simulink model "sdbe_8_11"  (R2012b)
settings: Solver=VariableStepDiscrete  SolverMode=SingleTasking  StartTime=0.0  StopTime=10000  RelTol=1e-3
PreLoadFcn:
  | counter_vals
undefined symbols (not defined in the file or in its folder): sfp
libraries: xbsIndex_r4 x6687, casper_library_misc x35, casper_library_delays x27, dspsigops x16, xps_library x10, r2dbe_vdif_lib x4, r2dbe_adc_lib x3, simulink x1
(part 1 of 58)
settings Model: Creator=lvertats  LastModifiedBy=lvertats
settings OptimizationCC: InlineParams=on

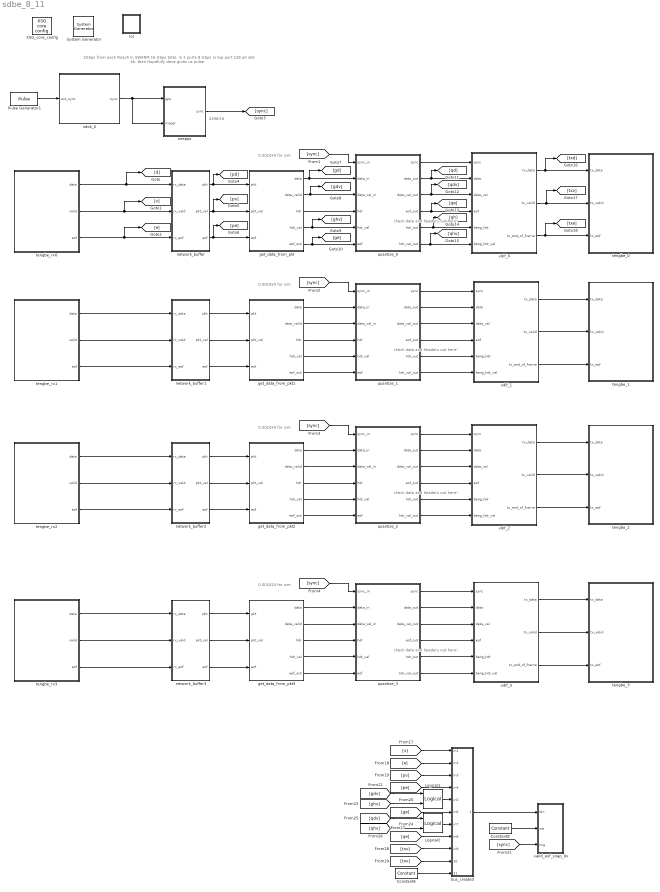
== system sdbe_8_11 ==
  note: 0.001024 for sim
  note: 2496/16
  note: check data and headers out here!
  note: 2Gbps from each Roach in SWARM
      | 16 Gbps total, in 2 ports
      | 8 Gbps in top port
      | 128 p0 sb0 4b, then
      |
      | Hopefully dave gives us pulse
  note: 0.001024 for sim
  note: check data and headers out here!
  note: 0.001024 for sim
  note: check data and headers out here!
  note: 0.001024 for sim
  note: check data and headers out here!
  " System Generator" : xbsIndex_r4/ System Generator  Tag=genX  xilinxfamily=virtex6  part=xc6vsx475t  speed=-1  package=ff1759  synthesis_tool=XST  clock_wrapper=Clock Enables  directory=./sdbe_8_11/sysgen  proj_type=Project Navigator  Synth_file=XST Defaults  Impl_file=ISE Defaults  testbench=off  simulink_period=1  sysclk_period=4.8077  dcm_input_clock_period=100  incr_netlist=off  trim_vbits=Everywhere in SubSystem  dbl_ovrd=According to Block Masks  core_generation=According to Block Masks  run_coregen=off  deprecated_control=off  eval_field=0  block_type=sysgen
  Constant6 : xbsIndex_r4/Constant  const=0  gui_display_data_type=Fixed-point  arith_type=Unsigned  n_bits=6  bin_pt=0  preci_type=Single  exp_width=8  frac_width=24  explicit_period=on  period=1  equ=P=C  opselect=C  inp2=PCIN>>17  opr=+  inp1=P  carry=CIN  dbl_ovrd=off  block_type=constant
  Constant8 : xbsIndex_r4/Constant  const=1  gui_display_data_type=Boolean  arith_type=Boolean  n_bits=31  bin_pt=0  preci_type=Single  exp_width=8  frac_width=24  explicit_period=on  period=1  equ=P=C  opselect=C  inp2=PCIN>>17  opr=+  inp1=P  carry=CIN  dbl_ovrd=off  block_type=constant
  Logical1 : xbsIndex_r4/Logical  logical_function=OR  inputs=2  en=off  latency=0  precision=Full  arith_type=Unsigned  n_bits=16  bin_pt=0  align_bp=on  dbl_ovrd=off  block_type=logical
  Logical2 : xbsIndex_r4/Logical  logical_function=OR  inputs=2  en=off  latency=0  precision=Full  arith_type=Unsigned  n_bits=16  bin_pt=0  align_bp=on  dbl_ovrd=off  block_type=logical
  Pulse Generator1 : DiscretePulseGenerator  Period=1024  PhaseDelay=57
  XSG_core_config : xps_library/XSG core config  Tag=xps:xsg  hw_sys=ROACH2:sx475t  clk_src=adc0_clk  ROACH_clk_src=sys_clk  ROACH2_clk_src=adc0_clk  MKDIG_clk_src=sys_clk  clk_rate=3328/16  sample_period=1  synthesis_tool=XST
  bus_create3 : Subsystem  AncestorBlock=casper_library_flow_control/bus_create  mask(bus_create){inputNum=11}
      mask prompts: inputNum "Number of inputs:"
      mask init:
      | bus_create_init(gcb,...
      |     'inputNum', inputNum);
  get_data_from_pkt : Subsystem
  get_data_from_pkt1 : Subsystem
  get_data_from_pkt2 : Subsystem
  get_data_from_pkt3 : Subsystem
  network_buffer : Subsystem
  network_buffer1 : Subsystem
  network_buffer2 : Subsystem
  network_buffer3 : Subsystem
  onepps : Subsystem  AncestorBlock=r2dbe_adc_lib/onepps  mask(r2dbe_onepps){clk_rate=3328/16}
      mask prompts: clk_rate "FPGA clock rate (MHz):"
      mask help: Sub-system for 1pps parameters of the R2DBE.
  quantize_0 : Subsystem  mask(r2dbe_quantize){mult_delay=3, add_delay=2, convert_delay=1, pipeline_delay=1, io_delay=3}
      mask prompts: mult_delay "Multiplier latency:"; add_delay "Adder latency:"; convert_delay "Convert latency:"; pipeline_delay "Output pipeline delay:"; io_delay "I/O delay:"
      mask help: Sub-system for quantization parameters of the R2DBE.
  quantize_1 : Subsystem  mask(r2dbe_quantize){mult_delay=3, add_delay=2, convert_delay=1, pipeline_delay=1, io_delay=3}
      mask prompts: mult_delay "Multiplier latency:"; add_delay "Adder latency:"; convert_delay "Convert latency:"; pipeline_delay "Output pipeline delay:"; io_delay "I/O delay:"
      mask help: Sub-system for quantization parameters of the R2DBE.
  quantize_2 : Subsystem  mask(r2dbe_quantize){mult_delay=3, add_delay=2, convert_delay=1, pipeline_delay=1, io_delay=3}
      mask prompts: mult_delay "Multiplier latency:"; add_delay "Adder latency:"; convert_delay "Convert latency:"; pipeline_delay "Output pipeline delay:"; io_delay "I/O delay:"
      mask help: Sub-system for quantization parameters of the R2DBE.
  quantize_3 : Subsystem  mask(r2dbe_quantize){mult_delay=3, add_delay=2, convert_delay=1, pipeline_delay=1, io_delay=3}
      mask prompts: mult_delay "Multiplier latency:"; add_delay "Adder latency:"; convert_delay "Convert latency:"; pipeline_delay "Output pipeline delay:"; io_delay "I/O delay:"
      mask help: Sub-system for quantization parameters of the R2DBE.
  rcs : Subsystem  AncestorBlock=casper_library_misc/rcs  mask(rcs){app_src=timestamp, lib_src=timestamp, user_val=0}
      mask prompts: app_src "Application revision info to capture"; lib_src "CASPER libraries revision info to capture"; user_val "User specified value"
      mask help:
      | Embeds revision control information for the user design and libraries.
      | On failure to locate specified revision information, falls back to
      | timestamps (current time for libraries).
      | A user specified value is also stored.
      mask init:
      | rcs_init(gcb, ...
      |     'app_src', app_src, ...
      |     'lib_src', lib_src);
      mask TypeOptions app_src: timestamp | git | svn
      mask TypeOptions lib_src: timestamp | git | svn
  tengbe_0 : Subsystem  mask(r2dbe_tengbe){slot=0, port=0}
      mask prompts: slot "Card slot:"
      mask help: Sub-system for 10 GbE parameters of the R2DBE.
      mask init:
      | set_param([gcb, '/core'], 'slot', slot);
      | set_param([gcb, '/core'], 'port_r2_sfpp', port);
      mask TypeOptions slot: 0 | 1
      mask TypeOptions port: 0 | 1 | 2 | 3
  tengbe_1 : Subsystem  mask(r2dbe_tengbe){slot=0, port=1}
      mask prompts: slot "Card slot:"
      mask help: Sub-system for 10 GbE parameters of the R2DBE.
      mask init:
      | set_param([gcb, '/core'], 'slot', slot);
      | set_param([gcb, '/core'], 'port_r2_sfpp', port);
      mask TypeOptions slot: 0 | 1
      mask TypeOptions port: 0 | 1 | 2 | 3
  tengbe_2 : Subsystem  mask(r2dbe_tengbe){slot=0, port=2}
      mask prompts: slot "Card slot:"
      mask help: Sub-system for 10 GbE parameters of the R2DBE.
      mask init:
      | set_param([gcb, '/core'], 'slot', slot);
      | set_param([gcb, '/core'], 'port_r2_sfpp', port);
      mask TypeOptions slot: 0 | 1
      mask TypeOptions port: 0 | 1 | 2 | 3
  tengbe_3 : Subsystem  mask(r2dbe_tengbe){slot=0, port=3}
      mask prompts: slot "Card slot:"
      mask help: Sub-system for 10 GbE parameters of the R2DBE.
      mask init:
      | set_param([gcb, '/core'], 'slot', slot);
      | set_param([gcb, '/core'], 'port_r2_sfpp', port);
      mask TypeOptions slot: 0 | 1
      mask TypeOptions port: 0 | 1 | 2 | 3
  tengbe_rx0 : Subsystem  mask(r2dbe_tengbe){slot=1, port=0}
      mask prompts: slot "Card slot:"
      mask help: Sub-system for 10 GbE parameters of the R2DBE.
      mask init:
      | set_param([gcb, '/core'], 'slot', slot);
      | set_param([gcb, '/core'], 'port_r2_sfpp', port);
      mask TypeOptions slot: 0 | 1
      mask TypeOptions port: 0 | 1 | 2 | 3
  tengbe_rx1 : Subsystem  mask(r2dbe_tengbe){slot=1, port=1}
      mask prompts: slot "Card slot:"
      mask help: Sub-system for 10 GbE parameters of the R2DBE.
      mask init:
      | set_param([gcb, '/core'], 'slot', slot);
      | set_param([gcb, '/core'], 'port_r2_sfpp', port);
      mask TypeOptions slot: 0 | 1
      mask TypeOptions port: 0 | 1 | 2 | 3
  tengbe_rx2 : Subsystem  mask(r2dbe_tengbe){slot=1, port=2}
      mask prompts: slot "Card slot:"
      mask help: Sub-system for 10 GbE parameters of the R2DBE.
      mask init:
      | set_param([gcb, '/core'], 'slot', slot);
      | set_param([gcb, '/core'], 'port_r2_sfpp', port);
      mask TypeOptions slot: 0 | 1
      mask TypeOptions port: 0 | 1 | 2 | 3
  tengbe_rx3 : Subsystem  mask(r2dbe_tengbe){slot=1, port=3}
      mask prompts: slot "Card slot:"
      mask help: Sub-system for 10 GbE parameters of the R2DBE.
      mask init:
      | set_param([gcb, '/core'], 'slot', slot);
      | set_param([gcb, '/core'], 'port_r2_sfpp', port);
      mask TypeOptions slot: 0 | 1
      mask TypeOptions port: 0 | 1 | 2 | 3
  valid_eof_snap_0x : Subsystem  Tag=casper:snapshot  AncestorBlock=casper_library_scopes/snapshot  mask(snapshot){storage=bram, dram_dimm=1, dram_clock=200, nsamples=14, data_width=16, offset=off, circap=off, value=off, use_dsp48=on}
      mask prompts: storage "Storage medium"; dram_dimm "DRAM dimm"; dram_clock "DRAM clock rate"; nsamples "Number of Samples (2^?)"; data_width "Data width"; offset "Start delay support"; circap "Circular capture support"; value "Extra value capture support"; use_dsp48 "Use DSP48s to implement counters"
      mask help:
      | Standard snap block, but with the following optional extras;
      |  1) Optionally delay the fabric trigger by a user-specified number of valids.
      |  2) Capture continuously after a trigger until a stop pulse is received. Data is captured into BRAM continuously, with old data being overwritten until a stop command is received. Then stop capturing when memory is filled. This enables you to get some data before and some data after the stop pulse. Use the 'tr_en_cnt' register to determine where you are in your vector. 'Addr' register's MSb now indicates 'busy capturing'.
      |  3) Optionally capture a value on an input port to a register at the same time as the first data sample.
      |  4) Implement counters using DSP48Es to save resources.
      mask init:
      | snapshot_init(gcb, ...
      |     'storage', storage, ...
      |     'dram_dimm', dram_dimm, ...
      |     'dram_clock', dram_clock, ...
      |     'nsamples', nsamples, ...
      |     'data_width', data_width, ...
      |     'offset', offset, ...
      |     'circap', circap, ...
      |     'value', value, ...
      |     'use_dsp48', use_dsp48);
      mask TypeOptions storage: bram | dram
      mask Callback storage: snapshot_callback();
      mask TypeOptions dram_dimm: 1 | 2 | 3 | 4
      mask TypeOptions dram_clock: 200 | 250 | 266 | 300 | 333
      mask TypeOptions data_width: 8 | 16 | 32 | 64 | 128
  vdif_0 : Subsystem  mask(r2dbe_vdif){}
      mask help: Sub-system for VDIF parameters of the R2DBE.
  vdif_1 : Subsystem  mask(r2dbe_vdif){}
      mask help: Sub-system for VDIF parameters of the R2DBE.
  vdif_2 : Subsystem  mask(r2dbe_vdif){}
      mask help: Sub-system for VDIF parameters of the R2DBE.
  vdif_3 : Subsystem  mask(r2dbe_vdif){}
      mask help: Sub-system for VDIF parameters of the R2DBE.
  zdok_0 : Subsystem  mask(r2dbe_zdok){zdok=ZDOK 0, nyquist_bw=1248, pipeline_delay=1}
      mask prompts: zdok "ADC board"; nyquist_bw "Nyquist bandwidth (MHz):"; pipeline_delay "Output pipeline delay:"
      mask help: Sub-system for ADC5g parameters of the R2DBE.
      mask init:
      | set_param([gcb, '/adc'], 'adc_brd', zdok);
      mask TypeOptions zdok: ZDOK 0 | ZDOK 1
  wires:
  vdif_0/1(tx_data) -> tengbe_0/1(tx_data), [txd]
  vdif_0/2(tx_valid) -> tengbe_0/2(tx_valid), [txv]
  vdif_0/3(tx_end_of_frame) -> [txe], tengbe_0/3(tx_eof)
  quantize_0/1(sync) -> vdif_0/1(sync)
  quantize_0/2(data_out) -> vdif_0/2(data), [qd]
  Pulse Generator1/1 -> zdok_0/1(ext_sync)
  zdok_0/1(sync) -> onepps/2(maser), onepps/1(gps)
  onepps/1(sync) -> [sync]
  quantize_0/3(data_val_out) -> vdif_0/3(data_val), [qdv]
  quantize_0/4(eof_out) -> vdif_0/4(eof), [qe]
  quantize_0/5(hdr_out) -> vdif_0/5(beng_hdr), [qh]
  quantize_0/6(hdr_val_out) -> vdif_0/6(beng_hdr_val), [qhv]
  network_buffer/1(pkt) -> [pd], get_data_from_pkt/1(pkt)
  network_buffer/2(pkt_val) -> [pv], get_data_from_pkt/2(pkt_val)
  network_buffer/3(eof) -> [pe], get_data_from_pkt/3(eof)
  get_data_from_pkt/5(eof_out) -> [ge], quantize_0/6(eof)
  get_data_from_pkt/4(hdr_val) -> [ghv], quantize_0/5(hdr_val)
  get_data_from_pkt/3(hdr) -> quantize_0/4(hdr)
  get_data_from_pkt/2(data_valid) -> [gdv], quantize_0/3(data_val_in)
  get_data_from_pkt/1(data) -> [gd], quantize_0/2(data_in)
  bus_create3/1(bus_out) -> valid_eof_snap_0x/1(din)
  Constant8/1 -> valid_eof_snap_0x/2(we)
  [sync] -> valid_eof_snap_0x/3(trig)
  [e] -> bus_create3/2(in2)
  [v] -> bus_create3/1(in1)
  [pv] -> bus_create3/3(in3)
  [pe] -> bus_create3/4(in4)
  Logical1/1 -> bus_create3/5(in5)
  [gdv] -> Logical1/1
  [ghv] -> Logical1/2
  [ge] -> bus_create3/6(in6)
  [qdv] -> Logical2/1
  [qhv] -> Logical2/2
  [qe] -> bus_create3/8(in8)
  Logical2/1 -> bus_create3/7(in7)
  [txv] -> bus_create3/9(in9)
  [txv] -> bus_create3/10(in10)
  Constant6/1 -> bus_create3/11(in11)
  tengbe_rx0/1(data) -> [d], network_buffer/1(rx_data)
  tengbe_rx0/2(valid) -> [v], network_buffer/2(rx_vald)
  tengbe_rx0/3(eof) -> [e], network_buffer/3(rx_eof)
  [sync] -> quantize_0/1(sync_in)
  quantize_1/1(sync) -> vdif_1/1(sync)
  quantize_1/2(data_out) -> vdif_1/2(data)
  quantize_1/3(data_val_out) -> vdif_1/3(data_val)
  quantize_1/4(eof_out) -> vdif_1/4(eof)
  quantize_1/5(hdr_out) -> vdif_1/5(beng_hdr)
  quantize_1/6(hdr_val_out) -> vdif_1/6(beng_hdr_val)
  network_buffer1/1(pkt) -> get_data_from_pkt1/1(pkt)
  network_buffer1/2(pkt_val) -> get_data_from_pkt1/2(pkt_val)
  network_buffer1/3(eof) -> get_data_from_pkt1/3(eof)
  get_data_from_pkt1/5(eof_out) -> quantize_1/6(eof)
  get_data_from_pkt1/4(hdr_val) -> quantize_1/5(hdr_val)
  get_data_from_pkt1/3(hdr) -> quantize_1/4(hdr)
  get_data_from_pkt1/2(data_valid) -> quantize_1/3(data_val_in)
  get_data_from_pkt1/1(data) -> quantize_1/2(data_in)
  tengbe_rx1/1(data) -> network_buffer1/1(rx_data)
  tengbe_rx1/2(valid) -> network_buffer1/2(rx_vald)
  tengbe_rx1/3(eof) -> network_buffer1/3(rx_eof)
  [sync] -> quantize_1/1(sync_in)
  quantize_2/1(sync) -> vdif_2/1(sync)
  quantize_2/2(data_out) -> vdif_2/2(data)
  quantize_2/3(data_val_out) -> vdif_2/3(data_val)
  quantize_2/4(eof_out) -> vdif_2/4(eof)
  quantize_2/5(hdr_out) -> vdif_2/5(beng_hdr)
  quantize_2/6(hdr_val_out) -> vdif_2/6(beng_hdr_val)
  network_buffer2/1(pkt) -> get_data_from_pkt2/1(pkt)
  network_buffer2/2(pkt_val) -> get_data_from_pkt2/2(pkt_val)
  network_buffer2/3(eof) -> get_data_from_pkt2/3(eof)
  get_data_from_pkt2/5(eof_out) -> quantize_2/6(eof)
  get_data_from_pkt2/4(hdr_val) -> quantize_2/5(hdr_val)
  get_data_from_pkt2/3(hdr) -> quantize_2/4(hdr)
  get_data_from_pkt2/2(data_valid) -> quantize_2/3(data_val_in)
  get_data_from_pkt2/1(data) -> quantize_2/2(data_in)
  tengbe_rx2/1(data) -> network_buffer2/1(rx_data)
  tengbe_rx2/2(valid) -> network_buffer2/2(rx_vald)
  tengbe_rx2/3(eof) -> network_buffer2/3(rx_eof)
  [sync] -> quantize_2/1(sync_in)
  quantize_3/1(sync) -> vdif_3/1(sync)
  quantize_3/2(data_out) -> vdif_3/2(data)
  quantize_3/3(data_val_out) -> vdif_3/3(data_val)
  quantize_3/4(eof_out) -> vdif_3/4(eof)
  quantize_3/5(hdr_out) -> vdif_3/5(beng_hdr)
  quantize_3/6(hdr_val_out) -> vdif_3/6(beng_hdr_val)
  network_buffer3/1(pkt) -> get_data_from_pkt3/1(pkt)
  network_buffer3/2(pkt_val) -> get_data_from_pkt3/2(pkt_val)
  network_buffer3/3(eof) -> get_data_from_pkt3/3(eof)
  get_data_from_pkt3/5(eof_out) -> quantize_3/6(eof)
  get_data_from_pkt3/4(hdr_val) -> quantize_3/5(hdr_val)
  get_data_from_pkt3/3(hdr) -> quantize_3/4(hdr)
  get_data_from_pkt3/2(data_valid) -> quantize_3/3(data_val_in)
  get_data_from_pkt3/1(data) -> quantize_3/2(data_in)
  tengbe_rx3/1(data) -> network_buffer3/1(rx_data)
  tengbe_rx3/2(valid) -> network_buffer3/2(rx_vald)
  tengbe_rx3/3(eof) -> network_buffer3/3(rx_eof)
  [sync] -> quantize_3/1(sync_in)
  vdif_1/3(tx_end_of_frame) -> tengbe_1/3(tx_eof)
  vdif_1/1(tx_data) -> tengbe_1/1(tx_data)
  vdif_1/2(tx_valid) -> tengbe_1/2(tx_valid)
  vdif_2/2(tx_valid) -> tengbe_2/2(tx_valid)
  vdif_2/3(tx_end_of_frame) -> tengbe_2/3(tx_eof)
  vdif_2/1(tx_data) -> tengbe_2/1(tx_data)
  vdif_3/2(tx_valid) -> tengbe_3/2(tx_valid)
  vdif_3/3(tx_end_of_frame) -> tengbe_3/3(tx_eof)
  vdif_3/1(tx_data) -> tengbe_3/1(tx_data)

== system sdbe_8_11/bus_create3 ==
  in1 : Inport
  in2 : Inport  Port=2
  in3 : Inport  Port=3
  in4 : Inport  Port=4
  in5 : Inport  Port=5
  in6 : Inport  Port=6
  in7 : Inport  Port=7
  in8 : Inport  Port=8
  in9 : Inport  Port=9
  in10 : Inport  Port=10
  in11 : Inport  Port=11
  concatenate : xbsIndex_r4/Concat  num_inputs=11  dbl_ovrd=off  block_type=concat
  reinterpret{1..11} (11 alike) : xbsIndex_r4/Reinterpret  force_arith_type=on  arith_type=Unsigned  force_bin_pt=on  bin_pt=0  block_type=reinterpret
      reinterpret1 settings: infoedit="Changes signal type without altering the binary representation.   You can changed the signal between signed and unsigned, and relocate the binary point.<br><br>Hardware notes: In hardware this block costs nothing.<br><br>Example:  Suppose the input is 6 bits wide, signed, with 2 fractional bits, and the output is forced to unsigned with 0 fractional bits.  Then an input of -2.0 (1110.00 in binary 2's complement) becomes an output of 56 (111000 in binary)."
      reinterpret2 settings: infoedit="Changes signal type without altering the binary representation.   You can changed the signal between signed and unsigned, and relocate the binary point.<br><br>Hardware notes: In hardware this block costs nothing.<br><br>Example:  Suppose the input is 6 bits wide, signed, with 2 fractional bits, and the output is forced to unsigned with 0 fractional bits.  Then an input of -2.0 (1110.00 in binary 2's complement) becomes an output of 56 (111000 in binary)."
  bus_out : Outport
  wires:
  concatenate/1 -> bus_out/1
  in1/1 -> reinterpret1/1
  reinterpret1/1 -> concatenate/1
  in2/1 -> reinterpret2/1
  reinterpret2/1 -> concatenate/2
  in3/1 -> reinterpret3/1
  reinterpret3/1 -> concatenate/3
  in4/1 -> reinterpret4/1
  reinterpret4/1 -> concatenate/4
  in5/1 -> reinterpret5/1
  reinterpret5/1 -> concatenate/5
  in6/1 -> reinterpret6/1
  reinterpret6/1 -> concatenate/6
  in7/1 -> reinterpret7/1
  reinterpret7/1 -> concatenate/7
  in8/1 -> reinterpret8/1
  reinterpret8/1 -> concatenate/8
  in9/1 -> reinterpret9/1
  reinterpret9/1 -> concatenate/9
  in10/1 -> reinterpret10/1
  reinterpret10/1 -> concatenate/10
  in11/1 -> reinterpret11/1
  reinterpret11/1 -> concatenate/11

== system sdbe_8_11/get_data_from_pkt ==
  note: can pass all through, but turn valid off for first
  pkt : Inport
  pkt_val : Inport  Port=2
  eof : Inport  Port=3
  Constant : Constant  Value=0
  Counter : xbsIndex_r4/Counter  cnt_type=Free Running  cnt_to=Inf  operation=Up  start_count=0  cnt_by_val=1  arith_type=Unsigned  n_bits=32  bin_pt=0  load_pin=off  rst=on  en=on  explicit_period=on  period=1  dbl_ovrd=off  use_behavioral_HDL=off  implementation=Fabric  block_type=counter
  Delay2 : xbsIndex_r4/Delay  rst=off  infoeditControl=Selection of Reset will increase slice count due to use of real FFs and instead of SRLs  en=off  latency=1  dbl_ovrd=off  reg_retiming=off  block_type=delay
  Delay3 : xbsIndex_r4/Delay  rst=off  infoeditControl=Selection of Reset will increase slice count due to use of real FFs and instead of SRLs  en=off  latency=1  dbl_ovrd=off  reg_retiming=off  block_type=delay
  Slice : xbsIndex_r4/Slice  nbits=1  boolean_output=on  mode=Upper Bit Location + Width  bit1=0  base1=MSB of Input  bit0=0  base0=LSB of Input  dbl_ovrd=off  block_type=slice
  Terminator : Terminator
  gen_valids1 : Subsystem
      mask help: latency 1
  npkts : Subsystem  Tag=xps:sw_reg  AncestorBlock=xps_library/software register  mask(swreg){mode=one value, io_dir=To Processor, io_delay=0, sample_period=1, names=reg, bitwidths=32, arith_types=0, bin_pts=0, sim_port=on, show_format=off}
      mask prompts: io_dir "I/O direction"; io_delay "I/O delay"; sample_period "Sample period"; names "Name:"; bitwidths "Bitwidth:"; arith_types "Type (ufix=0, fix=1, bool=2):"; bin_pts "Binary pt:"; sim_port "Provide sim input/output?"; show_format "Print format string?"
      mask init:
      | swreg_init(gcb)
      settings: AttributesFormatString=1output
      mask TypeOptions mode: one value | fields of equal size | fields of arbitrary size
      mask Callback mode: swreg_cb(gcb);
      mask TypeOptions io_dir: To Processor | From Processor
      mask Callback io_dir:
      | mask_enables = get_param(gcb, 'MaskEnables');
      | mask_names = get_param(gcb, 'MaskNames');
      | if strcmp(get_param(gcb, 'io_dir'), 'To Processor'),
      |     mask_enables{ismember(mask_names, 'sample_period')} = 'off';
      | else
      |     mask_enables{ismember(mask_names, 'sample_period')} = 'on';
      | end
      | set_param(gcb, 'MaskEnables', mask_enables);
      mask Callback bitwidths:
      | swreg_maskcheck(gcb);
      | % blk = gcb;
      | % mode = get_param(blk, 'mode');
      | % current_widths = eval(get_param(blk, 'bitwidths'));
      | % if (strcmp(mode, 'one value') || strcmp(mode, 'fields of equal size')) && (length(current_widths) > 1),
      | %     error('Only one width may be specified for this mode.');
      | % elseif strcmp(mode, 'fields of arbitrary size')
      | %     current_names = textscan(strtrim(strrep(strrep(get_param(blk, 'names'), ']', ''), '[', '')), '%s');
      | %     current_names = current_names{1};
      | %     numios = length(current_names);
      | %     if length(current_widths) ~= numios,
      | %         error('%d field names specified, but %d widths?', numios, length(current_widths));
      | %     end
      | % end
      | % total_width = 0;
      | % for ctr = 1 : length(current_widths),
      | %     total_width = total_width + current_widths(ctr);
      | % end
      | % if total_width > 32,
      | %     error('Total width must be 32 or less, set to %d.', total_width);
      | % end
      mask Callback arith_types:
      | [numios, ~, ~, ~, current_types] = swreg_maskcheck(gcb);
      | % blk = gcb;
      | % mode = get_param(blk, 'mode');
      | % current_types = eval(get_param(blk, 'arith_types'));
      | % numios = length(current_types);
      | % if (strcmp(mode, 'one value') || strcmp(mode, 'fields of equal size')) && (length(current_types) > 1),
      | %     error('Only one type may be specified for this mode.');
      | % elseif strcmp(mode, 'fields of arbitrary size')
      | %     current_names = textscan(strtrim(strrep(strrep(get_param(blk, 'names'), ']', ''), '[', '')), '%s');
      | %     current_names = current_names{1};
      | %     numios = length(current_names);
      | %     if length(current_types) ~= numios,
      | %         error('%d field names specified, but %d types?', numios, length(current_types));
      | %     end
      | % end
      | problem = 0;
      | for ctr = 1 : numios,
      |     t = current_types(ctr);
      |     if (t < 0) || (t > 2),
      |         problem = t;
      |         ctr = numios + 1;
      |     end
      | end
      | if problem ~= 0,
      |     error('Type cannot be %i, must be 0, 1 or 2.', problem);
      | end
      mask Callback bin_pts:
      | swreg_maskcheck(gcb);
      | % blk = gcb;
      | % mode = get_param(blk, 'mode');
      | % current_bins = eval(get_param(blk, 'bin_pts'));
      | % if (strcmp(mode, 'one value') || strcmp(mode, 'fields of equal size')) && (length(current_bins) > 1),
      | %     error('Only one binary pt may be specified for this mode.');
      | % elseif strcmp(mode, 'fields of arbitrary size')
      | %     current_names = textscan(strtrim(strrep(strrep(get_param(blk, 'names'), ']', ''), '[', '')), '%s');
      | %     current_names = current_names{1};
      | %     numios = length(current_names);
      | %     if length(current_bins) ~= numios,
      | %         error('%d field names specified, but %d binary pts?', numios, length(current_bins));
      | %     end
      | % end
  rst : Subsystem  Tag=xps:sw_reg  AncestorBlock=xps_library/software register  mask(swreg){mode=one value, io_dir=From Processor, io_delay=0, sample_period=1, names=reg, bitwidths=32, arith_types=0, bin_pts=0, sim_port=on, show_format=off}
      mask prompts: io_dir "I/O direction"; io_delay "I/O delay"; sample_period "Sample period"; names "Name:"; bitwidths "Bitwidth:"; arith_types "Type (ufix=0, fix=1, bool=2):"; bin_pts "Binary pt:"; sim_port "Provide sim input/output?"; show_format "Print format string?"
      mask init:
      | swreg_init(gcb)
      settings: AttributesFormatString=1input
      mask TypeOptions mode: one value | fields of equal size | fields of arbitrary size
      mask Callback mode: swreg_cb(gcb);
      mask TypeOptions io_dir: To Processor | From Processor
      mask Callback io_dir:
      | mask_enables = get_param(gcb, 'MaskEnables');
      | mask_names = get_param(gcb, 'MaskNames');
      | if strcmp(get_param(gcb, 'io_dir'), 'To Processor'),
      |     mask_enables{ismember(mask_names, 'sample_period')} = 'off';
      | else
      |     mask_enables{ismember(mask_names, 'sample_period')} = 'on';
      | end
      | set_param(gcb, 'MaskEnables', mask_enables);
      mask Callback bitwidths:
      | swreg_maskcheck(gcb);
      | % blk = gcb;
      | % mode = get_param(blk, 'mode');
      | % current_widths = eval(get_param(blk, 'bitwidths'));
      | % if (strcmp(mode, 'one value') || strcmp(mode, 'fields of equal size')) && (length(current_widths) > 1),
      | %     error('Only one width may be specified for this mode.');
      | % elseif strcmp(mode, 'fields of arbitrary size')
      | %     current_names = textscan(strtrim(strrep(strrep(get_param(blk, 'names'), ']', ''), '[', '')), '%s');
      | %     current_names = current_names{1};
      | %     numios = length(current_names);
      | %     if length(current_widths) ~= numios,
      | %         error('%d field names specified, but %d widths?', numios, length(current_widths));
      | %     end
      | % end
      | % total_width = 0;
      | % for ctr = 1 : length(current_widths),
      | %     total_width = total_width + current_widths(ctr);
      | % end
      | % if total_width > 32,
      | %     error('Total width must be 32 or less, set to %d.', total_width);
      | % end
      mask Callback arith_types:
      | [numios, ~, ~, ~, current_types] = swreg_maskcheck(gcb);
      | % blk = gcb;
      | % mode = get_param(blk, 'mode');
      | % current_types = eval(get_param(blk, 'arith_types'));
      | % numios = length(current_types);
      | % if (strcmp(mode, 'one value') || strcmp(mode, 'fields of equal size')) && (length(current_types) > 1),
      | %     error('Only one type may be specified for this mode.');
      | % elseif strcmp(mode, 'fields of arbitrary size')
      | %     current_names = textscan(strtrim(strrep(strrep(get_param(blk, 'names'), ']', ''), '[', '')), '%s');
      | %     current_names = current_names{1};
      | %     numios = length(current_names);
      | %     if length(current_types) ~= numios,
      | %         error('%d field names specified, but %d types?', numios, length(current_types));
      | %     end
      | % end
      | problem = 0;
      | for ctr = 1 : numios,
      |     t = current_types(ctr);
      |     if (t < 0) || (t > 2),
      |         problem = t;
      |         ctr = numios + 1;
      |     end
      | end
      | if problem ~= 0,
      |     error('Type cannot be %i, must be 0, 1 or 2.', problem);
      | end
      mask Callback bin_pts:
      | swreg_maskcheck(gcb);
      | % blk = gcb;
      | % mode = get_param(blk, 'mode');
      | % current_bins = eval(get_param(blk, 'bin_pts'));
      | % if (strcmp(mode, 'one value') || strcmp(mode, 'fields of equal size')) && (length(current_bins) > 1),
      | %     error('Only one binary pt may be specified for this mode.');
      | % elseif strcmp(mode, 'fields of arbitrary size')
      | %     current_names = textscan(strtrim(strrep(strrep(get_param(blk, 'names'), ']', ''), '[', '')), '%s');
      | %     current_names = current_names{1};
      | %     numios = length(current_names);
      | %     if length(current_bins) ~= numios,
      | %         error('%d field names specified, but %d binary pts?', numios, length(current_bins));
      | %     end
      | % end
  rx_output : Subsystem
  rx_output1 : Subsystem
  scope : Subsystem
  data : Outport
  data_valid : Outport  Port=2
  hdr : Outport  Port=3
  hdr_val : Outport  Port=4
  eof_out : Outport  Port=5
  wires:
  pkt/1 -> Delay2/1
  Delay2/1 -> [data], data/1, [hdr], hdr/1
  Delay3/1 -> [eof], eof_out/1
  eof/1 -> gen_valids1/2(eof), Delay3/1
  npkts/1(sim_out) -> Terminator/1
  Counter/1 -> npkts/1(out_reg)
  rst/1(in_reg) -> Slice/1
  Constant/1 -> rst/1(sim_1)
  Slice/1 -> Counter/1
  pkt_val/1 -> gen_valids1/1(pkt_val)
  gen_valids1/1(hdr_val) -> [hdr_val], hdr_val/1
  gen_valids1/2(data_val) -> [data_val], data_valid/1
  [eof] -> Counter/2
  [data_val] -> rx_output/2(val)
  [eof] -> rx_output/3(eof)
  [hdr_val] -> rx_output/1(sig)
  [data] -> rx_output1/3(data)
  [hdr] -> rx_output1/1(hdr)
  [hdr_val] -> rx_output1/2(hdr_val)
  [data_val] -> rx_output1/4(data_val)
  [data_val] -> scope/2(valid)
  [data] -> scope/1(data)

== system sdbe_8_11/get_data_from_pkt1 ==
  note: can pass all through, but turn valid off for first
  pkt : Inport
  pkt_val : Inport  Port=2
  eof : Inport  Port=3
  Constant : Constant  Value=0
  Counter : xbsIndex_r4/Counter  cnt_type=Free Running  cnt_to=Inf  operation=Up  start_count=0  cnt_by_val=1  arith_type=Unsigned  n_bits=32  bin_pt=0  load_pin=off  rst=on  en=on  explicit_period=on  period=1  dbl_ovrd=off  use_behavioral_HDL=off  implementation=Fabric  block_type=counter
  Delay2 : xbsIndex_r4/Delay  rst=off  infoeditControl=Selection of Reset will increase slice count due to use of real FFs and instead of SRLs  en=off  latency=1  dbl_ovrd=off  reg_retiming=off  block_type=delay
  Delay3 : xbsIndex_r4/Delay  rst=off  infoeditControl=Selection of Reset will increase slice count due to use of real FFs and instead of SRLs  en=off  latency=1  dbl_ovrd=off  reg_retiming=off  block_type=delay
  Slice : xbsIndex_r4/Slice  nbits=1  boolean_output=on  mode=Upper Bit Location + Width  bit1=0  base1=MSB of Input  bit0=0  base0=LSB of Input  dbl_ovrd=off  block_type=slice
  Terminator : Terminator
  gen_valids1 : Subsystem
      mask help: latency 1
  npkts : Subsystem  Tag=xps:sw_reg  AncestorBlock=xps_library/software register  mask(swreg){mode=one value, io_dir=To Processor, io_delay=0, sample_period=1, names=reg, bitwidths=32, arith_types=0, bin_pts=0, sim_port=on, show_format=off}
      mask prompts: io_dir "I/O direction"; io_delay "I/O delay"; sample_period "Sample period"; names "Name:"; bitwidths "Bitwidth:"; arith_types "Type (ufix=0, fix=1, bool=2):"; bin_pts "Binary pt:"; sim_port "Provide sim input/output?"; show_format "Print format string?"
      mask init:
      | swreg_init(gcb)
      settings: AttributesFormatString=1output
      mask TypeOptions mode: one value | fields of equal size | fields of arbitrary size
      mask Callback mode: swreg_cb(gcb);
      mask TypeOptions io_dir: To Processor | From Processor
      mask Callback io_dir:
      | mask_enables = get_param(gcb, 'MaskEnables');
      | mask_names = get_param(gcb, 'MaskNames');
      | if strcmp(get_param(gcb, 'io_dir'), 'To Processor'),
      |     mask_enables{ismember(mask_names, 'sample_period')} = 'off';
      | else
      |     mask_enables{ismember(mask_names, 'sample_period')} = 'on';
      | end
      | set_param(gcb, 'MaskEnables', mask_enables);
      mask Callback bitwidths:
      | swreg_maskcheck(gcb);
      | % blk = gcb;
      | % mode = get_param(blk, 'mode');
      | % current_widths = eval(get_param(blk, 'bitwidths'));
      | % if (strcmp(mode, 'one value') || strcmp(mode, 'fields of equal size')) && (length(current_widths) > 1),
      | %     error('Only one width may be specified for this mode.');
      | % elseif strcmp(mode, 'fields of arbitrary size')
      | %     current_names = textscan(strtrim(strrep(strrep(get_param(blk, 'names'), ']', ''), '[', '')), '%s');
      | %     current_names = current_names{1};
      | %     numios = length(current_names);
      | %     if length(current_widths) ~= numios,
      | %         error('%d field names specified, but %d widths?', numios, length(current_widths));
      | %     end
      | % end
      | % total_width = 0;
      | % for ctr = 1 : length(current_widths),
      | %     total_width = total_width + current_widths(ctr);
      | % end
      | % if total_width > 32,
      | %     error('Total width must be 32 or less, set to %d.', total_width);
      | % end
      mask Callback arith_types:
      | [numios, ~, ~, ~, current_types] = swreg_maskcheck(gcb);
      | % blk = gcb;
      | % mode = get_param(blk, 'mode');
      | % current_types = eval(get_param(blk, 'arith_types'));
      | % numios = length(current_types);
      | % if (strcmp(mode, 'one value') || strcmp(mode, 'fields of equal size')) && (length(current_types) > 1),
      | %     error('Only one type may be specified for this mode.');
      | % elseif strcmp(mode, 'fields of arbitrary size')
      | %     current_names = textscan(strtrim(strrep(strrep(get_param(blk, 'names'), ']', ''), '[', '')), '%s');
      | %     current_names = current_names{1};
      | %     numios = length(current_names);
      | %     if length(current_types) ~= numios,
      | %         error('%d field names specified, but %d types?', numios, length(current_types));
      | %     end
      | % end
      | problem = 0;
      | for ctr = 1 : numios,
      |     t = current_types(ctr);
      |     if (t < 0) || (t > 2),
      |         problem = t;
      |         ctr = numios + 1;
      |     end
      | end
      | if problem ~= 0,
      |     error('Type cannot be %i, must be 0, 1 or 2.', problem);
      | end
      mask Callback bin_pts:
      | swreg_maskcheck(gcb);
      | % blk = gcb;
      | % mode = get_param(blk, 'mode');
      | % current_bins = eval(get_param(blk, 'bin_pts'));
      | % if (strcmp(mode, 'one value') || strcmp(mode, 'fields of equal size')) && (length(current_bins) > 1),
      | %     error('Only one binary pt may be specified for this mode.');
      | % elseif strcmp(mode, 'fields of arbitrary size')
      | %     current_names = textscan(strtrim(strrep(strrep(get_param(blk, 'names'), ']', ''), '[', '')), '%s');
      | %     current_names = current_names{1};
      | %     numios = length(current_names);
      | %     if length(current_bins) ~= numios,
      | %         error('%d field names specified, but %d binary pts?', numios, length(current_bins));
      | %     end
      | % end
  rst : Subsystem  Tag=xps:sw_reg  AncestorBlock=xps_library/software register  mask(swreg){mode=one value, io_dir=From Processor, io_delay=0, sample_period=1, names=reg, bitwidths=32, arith_types=0, bin_pts=0, sim_port=on, show_format=off}
      mask prompts: io_dir "I/O direction"; io_delay "I/O delay"; sample_period "Sample period"; names "Name:"; bitwidths "Bitwidth:"; arith_types "Type (ufix=0, fix=1, bool=2):"; bin_pts "Binary pt:"; sim_port "Provide sim input/output?"; show_format "Print format string?"
      mask init:
      | swreg_init(gcb)
      settings: AttributesFormatString=1input
      mask TypeOptions mode: one value | fields of equal size | fields of arbitrary size
      mask Callback mode: swreg_cb(gcb);
      mask TypeOptions io_dir: To Processor | From Processor
      mask Callback io_dir:
      | mask_enables = get_param(gcb, 'MaskEnables');
      | mask_names = get_param(gcb, 'MaskNames');
      | if strcmp(get_param(gcb, 'io_dir'), 'To Processor'),
      |     mask_enables{ismember(mask_names, 'sample_period')} = 'off';
      | else
      |     mask_enables{ismember(mask_names, 'sample_period')} = 'on';
      | end
      | set_param(gcb, 'MaskEnables', mask_enables);
      mask Callback bitwidths:
      | swreg_maskcheck(gcb);
      | % blk = gcb;
      | % mode = get_param(blk, 'mode');
      | % current_widths = eval(get_param(blk, 'bitwidths'));
      | % if (strcmp(mode, 'one value') || strcmp(mode, 'fields of equal size')) && (length(current_widths) > 1),
      | %     error('Only one width may be specified for this mode.');
      | % elseif strcmp(mode, 'fields of arbitrary size')
      | %     current_names = textscan(strtrim(strrep(strrep(get_param(blk, 'names'), ']', ''), '[', '')), '%s');
      | %     current_names = current_names{1};
      | %     numios = length(current_names);
      | %     if length(current_widths) ~= numios,
      | %         error('%d field names specified, but %d widths?', numios, length(current_widths));
      | %     end
      | % end
      | % total_width = 0;
      | % for ctr = 1 : length(current_widths),
      | %     total_width = total_width + current_widths(ctr);
      | % end
      | % if total_width > 32,
      | %     error('Total width must be 32 or less, set to %d.', total_width);
      | % end
      mask Callback arith_types:
      | [numios, ~, ~, ~, current_types] = swreg_maskcheck(gcb);
      | % blk = gcb;
      | % mode = get_param(blk, 'mode');
      | % current_types = eval(get_param(blk, 'arith_types'));
      | % numios = length(current_types);
      | % if (strcmp(mode, 'one value') || strcmp(mode, 'fields of equal size')) && (length(current_types) > 1),
      | %     error('Only one type may be specified for this mode.');
      | % elseif strcmp(mode, 'fields of arbitrary size')
      | %     current_names = textscan(strtrim(strrep(strrep(get_param(blk, 'names'), ']', ''), '[', '')), '%s');
      | %     current_names = current_names{1};
      | %     numios = length(current_names);
      | %     if length(current_types) ~= numios,
      | %         error('%d field names specified, but %d types?', numios, length(current_types));
      | %     end
      | % end
      | problem = 0;
      | for ctr = 1 : numios,
      |     t = current_types(ctr);
      |     if (t < 0) || (t > 2),
      |         problem = t;
      |         ctr = numios + 1;
      |     end
      | end
      | if problem ~= 0,
      |     error('Type cannot be %i, must be 0, 1 or 2.', problem);
      | end
      mask Callback bin_pts:
      | swreg_maskcheck(gcb);
      | % blk = gcb;
      | % mode = get_param(blk, 'mode');
      | % current_bins = eval(get_param(blk, 'bin_pts'));
      | % if (strcmp(mode, 'one value') || strcmp(mode, 'fields of equal size')) && (length(current_bins) > 1),
      | %     error('Only one binary pt may be specified for this mode.');
      | % elseif strcmp(mode, 'fields of arbitrary size')
      | %     current_names = textscan(strtrim(strrep(strrep(get_param(blk, 'names'), ']', ''), '[', '')), '%s');
      | %     current_names = current_names{1};
      | %     numios = length(current_names);
      | %     if length(current_bins) ~= numios,
      | %         error('%d field names specified, but %d binary pts?', numios, length(current_bins));
      | %     end
      | % end
  rx_output : Subsystem
  rx_output1 : Subsystem
  scope : Subsystem
  data : Outport
  data_valid : Outport  Port=2
  hdr : Outport  Port=3
  hdr_val : Outport  Port=4
  eof_out : Outport  Port=5
  wires:
  [data] -> scope/1(data)
  [data_val] -> scope/2(valid)
  [data_val] -> rx_output1/4(data_val)
  [hdr_val] -> rx_output1/2(hdr_val)
  [hdr] -> rx_output1/1(hdr)
  [data] -> rx_output1/3(data)
  [hdr_val] -> rx_output/1(sig)
  [eof] -> rx_output/3(eof)
  [data_val] -> rx_output/2(val)
  [eof] -> Counter/2
  gen_valids1/2(data_val) -> data_valid/1, [data_val]
  gen_valids1/1(hdr_val) -> hdr_val/1, [hdr_val]
  pkt_val/1 -> gen_valids1/1(pkt_val)
  Slice/1 -> Counter/1
  Constant/1 -> rst/1(sim_1)
  rst/1(in_reg) -> Slice/1
  Counter/1 -> npkts/1(out_reg)
  npkts/1(sim_out) -> Terminator/1
  eof/1 -> Delay3/1, gen_valids1/2(eof)
  Delay3/1 -> eof_out/1, [eof]
  Delay2/1 -> hdr/1, [hdr], data/1, [data]
  pkt/1 -> Delay2/1
